simulink model "MARS"  (R2022a)
settings: Solver=VariableStepAuto  StartTime=0.0  StopTime=inf  RelTol=1e-3
model workspace (MAT data in the model file):
  T0 = -23.4
  h_trop = 7
  ingenuityParams.environment.gravity = -3.721
  ingenuityParams.environment.atmDensity = 0.01
  ingenuityParams.mechanical.totalMassExceptBatteries = 1.5
  ingenuityParams.propeller.diameter = 1.2
  ingenuityParams.propeller.inertia = 0.0042
  ingenuityParams.propeller.Jvec = [-0.8 -0.6 -0.4 -0.2 0 0.2 0.4 0.6 0.8 1]
  ingenuityParams.propeller.kTvec = [-0.02 0.02 0.06 0.09 0.12 0.1 0.08 0.05 0 -0.03]
  ingenuityParams.propeller.kPvec = [0.018 0.044 0.055 0.053 0.05 0.051 0.052 0.04 0.015 -0.01]
  ingenuityParams.motordrive.torMax = 0.25
  ingenuityParams.motordrive.powMax = 350
  ingenuityParams.motordrive.Tc = 0.01
  ingenuityParams.motordrive.effRated = 95
  ingenuityParams.motordrive.wRated = 12000
  ingenuityParams.motordrive.torRated = 0.15
  ingenuityParams.motordrive.ironLoss = 1
  ingenuityParams.motordrive.fixedLoss = 0.1
  ingenuityParams.motordrive.supplyRes = 0.07
  ingenuityParams.gearbox.ratio = 5
  ingenuityParams.battery.numSeriesCells = 6
  ingenuityParams.battery.numParallelStrings = 1
  ingenuityParams.battery.numCells = 6
  ingenuityParams.battery.cell.SOCvec = [0 0.01 0.02 0.03 0.04 0.05 0.06 0.07 0.08 0.09 0.1 0.11 0.12 0.13 0.14 0.15 0.16 0.17 0.18 0.19 0.2 0.21 0.22 0.23 0.24 0.25 0.26 0.27 0.28 0.29 0.3 0.31 0.32 0.33 0.34 0.35 0.36 0.37 0.38 0.39 0.4 0.41 0.42 0.43 0.44 0.45 0.46 0.47 0.48 0.49 0.5 0.51 0.52 0.53 0.54 0.55 0.56 0.57 0.58 0.59 0.6 0.61 0.62 0.63 0.64 0.65 0.66 0.67 0.68 0.69 0.7 0.71 0.72 0.73 0.74 0.75 0.76 0.77 0.78 0.79 0.8 0.81 0.82 0.83 0.84 0.85 0.86 0.87 0.88 0.89 0.9 0.91 0.92 0.93 0.94 0.95 0.96 0.97 0.98 0.99 1]
  ingenuityParams.battery.cell.Tvec = [-20 -10 0 20 40]
  ingenuityParams.battery.cell.V0_TLU = [3.43105105188 3.58415322084 3.62260441789 3.64734185538 3.64653306426 3.65558876806 3.66332769116 3.66323970813 3.66627838389 3.66945052656 3.67178851676 3.6762818022 ... (505 elements, 101x5)]
  ingenuityParams.battery.cell.R0_TLU = [0.0677427338002 0.0762862248111 0.0765216743797 0.0757633732548 0.0731538961444 0.0712592375055 0.0700448036528 0.0683159100683 0.0668135859615 0.0653209333694 0.0637678349468 0.0623709173386 ... (505 elements, 101x5)]
  ingenuityParams.battery.cell.AH_TLU = [0.302116721618 0.361031685699 0.377020499472 0.396021549816 0.399328545287]
  ingenuityParams.battery.cell.mass = 0.07
  ingenuityParams.battery.cell.cp = 500
  ingenuityParams.battery.cell.T_init = -16
  ingenuityParams.battery.cell.SOC_init = 0.99
  ingenuityParams.battery.thermal.cell2cellCond.area = 0.0001
  ingenuityParams.battery.thermal.cell2cellCond.thick = 0.01
  ingenuityParams.battery.thermal.cell2cellCond.k = 200
  ingenuityParams.battery.thermal.radToBox.area = 0.00628318530718
  ingenuityParams.battery.thermal.radToBox.radCoeff = 3.969e-08
  ingenuityParams.battery.thermal.insulationLayer.area = 0.24
  ingenuityParams.battery.thermal.insulationLayer.thick = 0.005
  ingenuityParams.battery.thermal.insulationLayer.k = 0.02
  ingenuityParams.battery.thermal.insulantThermalMass.mass = 0.03
  ingenuityParams.battery.thermal.insulantThermalMass.cp = 1200
  ingenuityParams.battery.thermal.radToEnvironment.area = 0.24
  ingenuityParams.battery.thermal.radToEnvironment.radCoeff = 1.701e-08
  ingenuityParams.heater.R = 40
  ingenuityParams.heater.thermalMass = 9
  ingenuityParams.solarcells.Isc = 0.15
  ingenuityParams.solarcells.Voc = 0.85
  ingenuityParams.solarcells.Ir0 = 500
  ingenuityParams.solarcells.qualFactor = 1.5
  ingenuityParams.solarcells.Rs = 0
  ingenuityParams.solarcells.Nseries = 30
  ingenuityParams.solarcells.Nparallel = 1
undefined symbols (not defined in the file): body, collective1, collective2, duration, ingenuity, leg1, leg2, leg3, leg4, link_name, model_name, rotor1, rotor2, solarPanel, world_pose
libraries: fl_lib x35, robotgazebolib x31, nesl_utility x12, ee_lib x11, slpidlib x3, sharedtransform x2, simulink x1, shared6dof x1, aerolibwind2 x1
(part 1 of 3)
settings Model: Creator=aman  LastModifiedBy=aman
settings SolverCC: MaxConsecutiveMinStep=2  ZeroCrossAlgorithm=Adaptive
settings OptimizationCC: DefaultParameterBehavior=Inlined  UseDivisionForNetSlopeComputation=on  GainParamInheritBuiltInType=on  UseFloatMulNetSlope=on  InlineInvariantSignals=on  EfficientFloat2IntCast=on
settings DebuggingCC: IgnoredZcDiagnostic=none
settings HardwareCC: TargetBitPerLong=64  TargetBitPerPointer=64  TargetBitPerSizeT=64  TargetBitPerPtrDiffT=64  TargetLongLongMode=on  TargetIntDivRoundTo=Zero  TargetEndianess=LittleEndian  TargetWordSize=64  TargetHWDeviceType=MATLAB Host  ProdEqTarget=off
settings SFSimCC: MATLABDynamicMemAlloc=off  SimHardwareAcceleration=native  SimTargetLang=C++
settings RTWCC: Description=Rapid Simulation Target  SystemTargetFile=rsim.tlc  TemplateMakefile=rsim_default_tmf  GenerateReport=on  BuildConfiguration=Faster Runs  LaunchReport=on
settings CodeAppCC: ForceParamTrailComments=on
settings RSimTargetCC: TargetLangStandard=C99 (ISO)  OptimizeReductions=off
settings SimscapeCC: SimscapeLogType=all

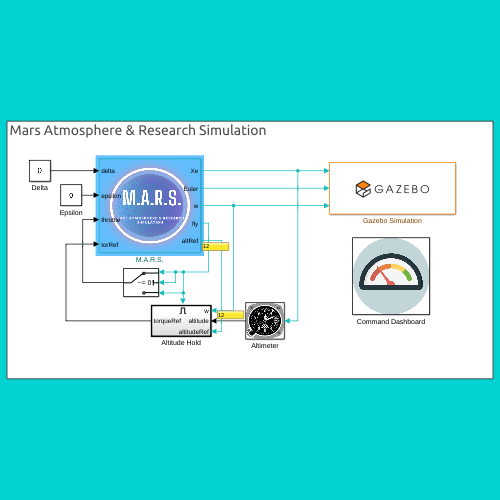
[thumbnail: Simulink's stored preview of the top-level diagram]
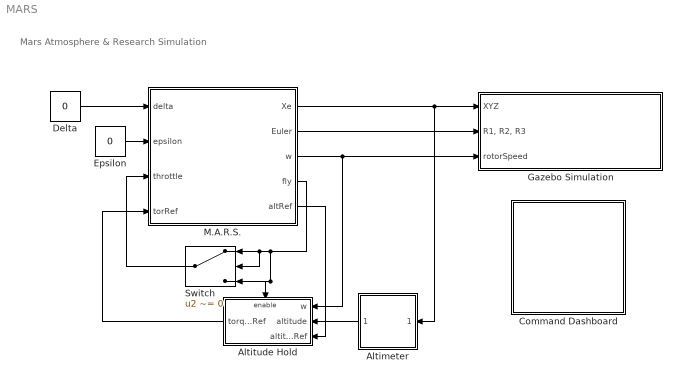
== system MARS ==
  note: Mars Atmosphere & Research Simulation
  Altimeter : Subsystem
      mask Display: image('$imagefile'); % Use "Edit Image" on toolstrip to change.
  Altitude Hold : Subsystem  TreatAsAtomicUnit=on
  Command Dashboard : Subsystem
      mask Display: image('$imagefile'); % Use "Edit Image" on toolstrip to change.
  Delta : Constant  Value=0
  Epsilon : Constant  Value=0
  Gazebo Simulation : Subsystem
      mask Display: image('$imagefile'); % Use "Edit Image" on toolstrip to change.
  M.A.R.S. : Subsystem
      mask Display: image('/home/aman/Desktop/mars.png'); % Use "Edit Image" on toolstrip to change.
  Switch : Switch  Criteria=u2 ~= 0  SaturateOnIntegerOverflow=off  InputSameDT=off
  wires:
  Delta/1 -> M.A.R.S./1(delta)
  Epsilon/1 -> M.A.R.S./2(epsilon)
  M.A.R.S./1(Xe) -> Gazebo Simulation/1(XYZ), Altimeter/1(height)
  Altimeter/1(altitude) -> Altitude Hold/2(altitude)
  M.A.R.S./3(w) -> Gazebo Simulation/3(rotorSpeed), Altitude Hold/1(w)
  Altitude Hold/1(torqueRef) -> M.A.R.S./4(torRef)
  M.A.R.S./5(altRef) -> Altitude Hold/3(altitudeRef)
  M.A.R.S./4(fly) -> Switch/3, Altitude Hold/Enable, Switch/2, Switch/1
  Switch/1 -> M.A.R.S./3(throttle)
  M.A.R.S./2(Euler) -> Gazebo Simulation/2("R1, R2, R3")

== system MARS/Altimeter ==
  height : Inport
  Band-Limited White Noise : simulink/Sources/Band-Limited White Noise  Cov=[0.1]  Ts=0.1  seed=[23341]
  Constant : Constant  Value=0
  Height : MultiPortSwitch  Inputs=1  SaturateOnIntegerOverflow=off  InputSameDT=off
  Index : Constant  Value=3
  Sum : Sum  Inputs=|++
  altitude : Outport
  wires:
  height/1 -> Height/2
  Height/1 -> Sum/2
  Index/1 -> Height/1
  Sum/1 -> altitude/1
  Constant/1 -> Sum/1

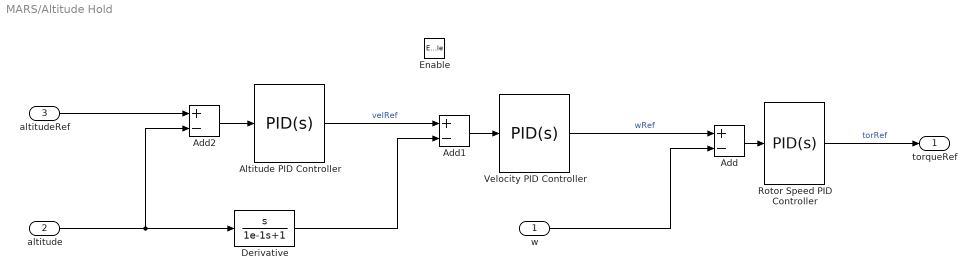
== system MARS/Altitude Hold ==
  w : Inport
  altitude : Inport  Port=2
  altitudeRef : Inport  Port=3
  Enable : EnablePort
  Add : Sum  Inputs=+-
  Add1 : Sum  Inputs=+-
  Add2 : Sum  Inputs=+-
  Altitude PID Controller : slpidlib/PID Controller  Controller=PID  Form=Parallel  TimeDomain=Continuous-time  UseExternalTs=off  SampleTime=-1  IntegratorMethod=Forward Euler  FilterMethod=Forward Euler  ControllerParametersSource=internal  P=2.75291380025279  I=0.654733901603954  UseKiTs=off  D=2.09643844624086  N=374.082600822232  UseFilter=on  TunerSelectOption=Transfer Function Based (PID Tuner App)  ZeroCross=off  InitialConditionSource=internal  InitialConditionForIntegrator=0  InitialConditionForFilter=0  DifferentiatorICPrevScaledInput=0  ExternalReset=none  TrackingMode=off  Kt=1  LimitOutput=on  SatLimitsSource=internal  UpperSaturationLimit=3  LowerSaturationLimit=-3  LinearizeAsGain=off  AntiWindupMode=clamping  Kb=1  POutMin=[]  POutMax=[]  IOutMin=[]  IOutMax=[]  DOutMin=[]  DOutMax=[]  NOutMin=[]  NOutMax=[]  SumOutMin=[]  SumOutMax=[]  SaturationOutMin=[]  SaturationOutMax=[]  PParamMin=[]  PParamMax=[]  IParamMin=[]  IParamMax=[]  DParamMin=[]  DParamMax=[]  NParamMin=[]  NParamMax=[]  KbParamMin=[]  KbParamMax=[]  KtParamMin=[]  KtParamMax=[]  KbOutMin=[]  KbOutMax=[]  KtOutMin=[]  KtOutMax=[]  IntegratorOutMin=[]  IntegratorOutMax=[]  FilterOutMin=[]  FilterOutMax=[]  SumI1OutMin=[]  SumI1OutMax=[]  SumI2OutMin=[]  SumI2OutMax=[]  SumI3OutMin=[]  SumI3OutMax=[]  SumI4OutMin=[]  SumI4OutMax=[]  SumDOutMin=[]  SumDOutMax=[]  DifferentiatorOutMin=[]  DifferentiatorOutMax=[]  FilterDiffOutCoefMin=[]  FilterDiffOutCoefMax=[]  ReciprocalOutMin=[]  ReciprocalOutMax=[]  SumDenOutMin=[]  SumDenOutMax=[]  SumNumOutMin=[]  SumNumOutMax=[]  DivideOutMin=[]  DivideOutMax=[]  UdiffTsProdOutMin=[]  UdiffTsProdOutMax=[]  NTsProdOutMin=[]  NTsProdOutMax=[]  UintegralTsProdOutMin=[]  UintegralTsProdOutMax=[]  UngainTsProdOutMin=[]  UngainTsProdOutMax=[]  IntegratorContinuousStateAttributes=''  IntegratorStateMustResolveToSignalObject=off  IntegratorRTWStateStorageClass=Auto  FilterContinuousStateAttributes=''  FilterStateMustResolveToSignalObject=off  FilterRTWStateStorageClass=Auto  ParallelPVariant=InternalParameters  IdealPVariant=Disabled  IVariant=InternalParameters  DVariant=InternalParameters  IntegratorVariant=Continuous  SatVariant=Enabled  AWVariant=ContClampingParallel  PCopyVariant=Disabled  TRVariant=Disabled  FdbkBlocksVariant=Forward  IdealPFdbkVariant=Disabled  SatFdbkVariant=Disabled  DerivativeFilterVariant=ContFilter  NVariant=InternalParameters  NCopyVariant=Disabled  FilterICVariant=InternalICsFilter  IntegratorICVariant=InternalICs  ExternalResetVariant=Disabled  TRSumVariant=Passthrough  SumFdbkVariant=Disabled  SumVariant=Sum_PID  TsampFilterVariant=InternalTs  TsampNgainVariant=Passthrough  TsampIntegralVariant=Passthrough  ExternalSaturationOutDataTypeStr=Inherit: Same as second input  aMode=0
  Derivative : TransferFcn  Numerator=[1 0]  Denominator=[1e-1 1]
  Rotor Speed PID Controller : slpidlib/PID Controller  Controller=PID  Form=Parallel  TimeDomain=Continuous-time  UseExternalTs=off  SampleTime=-1  IntegratorMethod=Forward Euler  FilterMethod=Forward Euler  ControllerParametersSource=internal  P=0.0108155264440049  I=0.00620055806015913  UseKiTs=off  D=0.000544690366654068  N=7717.3085682068  UseFilter=on  TunerSelectOption=Transfer Function Based (PID Tuner App)  ZeroCross=off  InitialConditionSource=internal  InitialConditionForIntegrator=0  InitialConditionForFilter=0  DifferentiatorICPrevScaledInput=0  ExternalReset=none  TrackingMode=off  Kt=1  LimitOutput=on  SatLimitsSource=internal  UpperSaturationLimit=0.3  LowerSaturationLimit=-0.3  LinearizeAsGain=off  AntiWindupMode=clamping  Kb=1  POutMin=[]  POutMax=[]  IOutMin=[]  IOutMax=[]  DOutMin=[]  DOutMax=[]  NOutMin=[]  NOutMax=[]  SumOutMin=[]  SumOutMax=[]  SaturationOutMin=[]  SaturationOutMax=[]  PParamMin=[]  PParamMax=[]  IParamMin=[]  IParamMax=[]  DParamMin=[]  DParamMax=[]  NParamMin=[]  NParamMax=[]  KbParamMin=[]  KbParamMax=[]  KtParamMin=[]  KtParamMax=[]  KbOutMin=[]  KbOutMax=[]  KtOutMin=[]  KtOutMax=[]  IntegratorOutMin=[]  IntegratorOutMax=[]  FilterOutMin=[]  FilterOutMax=[]  SumI1OutMin=[]  SumI1OutMax=[]  SumI2OutMin=[]  SumI2OutMax=[]  SumI3OutMin=[]  SumI3OutMax=[]  SumI4OutMin=[]  SumI4OutMax=[]  SumDOutMin=[]  SumDOutMax=[]  DifferentiatorOutMin=[]  DifferentiatorOutMax=[]  FilterDiffOutCoefMin=[]  FilterDiffOutCoefMax=[]  ReciprocalOutMin=[]  ReciprocalOutMax=[]  SumDenOutMin=[]  SumDenOutMax=[]  SumNumOutMin=[]  SumNumOutMax=[]  DivideOutMin=[]  DivideOutMax=[]  UdiffTsProdOutMin=[]  UdiffTsProdOutMax=[]  NTsProdOutMin=[]  NTsProdOutMax=[]  UintegralTsProdOutMin=[]  UintegralTsProdOutMax=[]  UngainTsProdOutMin=[]  UngainTsProdOutMax=[]  IntegratorContinuousStateAttributes=''  IntegratorStateMustResolveToSignalObject=off  IntegratorRTWStateStorageClass=Auto  FilterContinuousStateAttributes=''  FilterStateMustResolveToSignalObject=off  FilterRTWStateStorageClass=Auto  ParallelPVariant=InternalParameters  IdealPVariant=Disabled  IVariant=InternalParameters  DVariant=InternalParameters  IntegratorVariant=Continuous  SatVariant=Enabled  AWVariant=ContClampingParallel  PCopyVariant=Disabled  TRVariant=Disabled  FdbkBlocksVariant=Forward  IdealPFdbkVariant=Disabled  SatFdbkVariant=Disabled  DerivativeFilterVariant=ContFilter  NVariant=InternalParameters  NCopyVariant=Disabled  FilterICVariant=InternalICsFilter  IntegratorICVariant=InternalICs  ExternalResetVariant=Disabled  TRSumVariant=Passthrough  SumFdbkVariant=Disabled  SumVariant=Sum_PID  TsampFilterVariant=InternalTs  TsampNgainVariant=Passthrough  TsampIntegralVariant=Passthrough  ExternalSaturationOutDataTypeStr=Inherit: Same as second input  aMode=0
  Velocity PID Controller : slpidlib/PID Controller  Controller=PID  Form=Parallel  TimeDomain=Continuous-time  UseExternalTs=off  SampleTime=-1  IntegratorMethod=Forward Euler  FilterMethod=Forward Euler  ControllerParametersSource=internal  P=155.19306060889  I=41.1553609138668  UseKiTs=off  D=46.7041807942439  N=1.30346385486406  UseFilter=on  TunerSelectOption=Transfer Function Based (PID Tuner App)  ZeroCross=off  InitialConditionSource=internal  InitialConditionForIntegrator=0  InitialConditionForFilter=0  DifferentiatorICPrevScaledInput=0  ExternalReset=none  TrackingMode=off  Kt=1  LimitOutput=on  SatLimitsSource=internal  UpperSaturationLimit=1600  LowerSaturationLimit=0  LinearizeAsGain=off  AntiWindupMode=clamping  Kb=1  POutMin=[]  POutMax=[]  IOutMin=[]  IOutMax=[]  DOutMin=[]  DOutMax=[]  NOutMin=[]  NOutMax=[]  SumOutMin=[]  SumOutMax=[]  SaturationOutMin=[]  SaturationOutMax=[]  PParamMin=[]  PParamMax=[]  IParamMin=[]  IParamMax=[]  DParamMin=[]  DParamMax=[]  NParamMin=[]  NParamMax=[]  KbParamMin=[]  KbParamMax=[]  KtParamMin=[]  KtParamMax=[]  KbOutMin=[]  KbOutMax=[]  KtOutMin=[]  KtOutMax=[]  IntegratorOutMin=[]  IntegratorOutMax=[]  FilterOutMin=[]  FilterOutMax=[]  SumI1OutMin=[]  SumI1OutMax=[]  SumI2OutMin=[]  SumI2OutMax=[]  SumI3OutMin=[]  SumI3OutMax=[]  SumI4OutMin=[]  SumI4OutMax=[]  SumDOutMin=[]  SumDOutMax=[]  DifferentiatorOutMin=[]  DifferentiatorOutMax=[]  FilterDiffOutCoefMin=[]  FilterDiffOutCoefMax=[]  ReciprocalOutMin=[]  ReciprocalOutMax=[]  SumDenOutMin=[]  SumDenOutMax=[]  SumNumOutMin=[]  SumNumOutMax=[]  DivideOutMin=[]  DivideOutMax=[]  UdiffTsProdOutMin=[]  UdiffTsProdOutMax=[]  NTsProdOutMin=[]  NTsProdOutMax=[]  UintegralTsProdOutMin=[]  UintegralTsProdOutMax=[]  UngainTsProdOutMin=[]  UngainTsProdOutMax=[]  IntegratorContinuousStateAttributes=''  IntegratorStateMustResolveToSignalObject=off  IntegratorRTWStateStorageClass=Auto  FilterContinuousStateAttributes=''  FilterStateMustResolveToSignalObject=off  FilterRTWStateStorageClass=Auto  ParallelPVariant=InternalParameters  IdealPVariant=Disabled  IVariant=InternalParameters  DVariant=InternalParameters  IntegratorVariant=Continuous  SatVariant=Enabled  AWVariant=ContClampingParallel  PCopyVariant=Disabled  TRVariant=Disabled  FdbkBlocksVariant=Forward  IdealPFdbkVariant=Disabled  SatFdbkVariant=Disabled  DerivativeFilterVariant=ContFilter  NVariant=InternalParameters  NCopyVariant=Disabled  FilterICVariant=InternalICsFilter  IntegratorICVariant=InternalICs  ExternalResetVariant=Disabled  TRSumVariant=Passthrough  SumFdbkVariant=Disabled  SumVariant=Sum_PID  TsampFilterVariant=InternalTs  TsampNgainVariant=Passthrough  TsampIntegralVariant=Passthrough  ExternalSaturationOutDataTypeStr=Inherit: Same as second input  aMode=0
  torqueRef : Outport  OutputWhenDisabled=reset  InitialOutput=0
  wires:
  Add2/1 -> Altitude PID Controller/1
  Rotor Speed PID Controller/1 -> torqueRef/1  "torRef"
  Add/1 -> Rotor Speed PID Controller/1
  Add1/1 -> Velocity PID Controller/1
  w/1 -> Add/2
  Velocity PID Controller/1 -> Add/1  "wRef"
  altitude/1 -> Add2/2, Derivative/1
  Derivative/1 -> Add1/2
  Altitude PID Controller/1 -> Add1/1  "velRef"
  altitudeRef/1 -> Add2/1

== system MARS/Command Dashboard ==
  note: Measurements and Controller State
  note: Martian Environment Variables & Controls
  Altimeter : AltimeterBlock
  Altitude [m] : LinearGaugeBlock  LabelPosition=Hide  ScaleMax=50  TickInterval=2
  Artificial Horizon : ArtificialHorizonBlock
  Battery SOC : CircularGaugeBlock  LabelPosition=Hide  ScaleMax=1  TickInterval=0.2
  "Battery Temperature [degC] " : SemiCircularGaugeBlock  LabelPosition=Hide  ScaleMin=-60  ScaleMax=40  TickInterval=20
  Flying : LampBlock  LabelPosition=Hide
  Heater On : LampBlock  LabelPosition=Hide
  Prepare Flight : ToggleSwitchBlock  LabelPosition=Hide
      settings: Values={{'Off', 'On'}, [0 1]}
  Solar Irradiation [W/m^2] : SliderBlock  LabelPosition=Hide  ScaleMax=500
  Surface Temperature [degC] : SliderBlock  LabelPosition=Hide  ScaleMin=-125  ScaleMax=50
  delta : CustomTuningWebBlock  LabelPosition=Hide  ShowInitialText=on  Configuration="{\"type\":\"LinearGauge\",\"settings\":{\"BindingType\":\"param\",\"aspectRatio\":3.7777777777777777,\"backgroundColor\":[0,0,0,\"1\"],\"backgroundOffset\":0,\"backgroundOpacity\":1,\"fixedAspectRatio\":\"on\",\"foregroundColor\":[252,252,196],\"orientation\":\"horizontal\",\"showBackgroundColor\":false,\"value\":0},\"components\":[{\"name\":\"LinearScaleComponent\",\"settings\":{\"bounds\":{\"max\":0.1,\"min\":-0.1,\"tickInterval\":\"auto\"},\"internalTickHeightScaleFactor\":0.5,\"labelColor\":[255,255,200],\"labelFont\":{\"font\":\"Arial\",\"fontSize\":12},\"labelTransparency\":1,\"needleImage\":{\"size\":[596,842],\"src\":\"data:image/svg+xml;base64,PD94bWwgdmVyc2lvbj0iMS4wIiBlbmNvZGluZz0idXRmLTgiPz4NCjwhLS0gR2VuZXJhdG9yOiBBZG9iZSBJbGx1c3RyYXRvciAyNS4wLjAsIFNWRyBFeHBvcnQgUGx1Zy1JbiAuIFNWRyBWZXJzaW9uOiA2LjAwIEJ1aWxkIDApICAtLT4NCjxzdmcgdmVyc2lvbj0iMS4xIg0KCSBpZD0ic3ZnOCIgeG1sbnM6Y2M9Imh0dHA6Ly9jcmVhdGl2ZWNvbW1vbnMub3JnL25zIyIgeG1sbnM6ZGM9Imh0dHA6Ly9wdXJsLm9yZy9kYy9lbGVtZW50cy8xLjEvIiB4bWxuczppbmtzY2FwZT0iaHR0cDovL3d3dy5pbmtzY2FwZS5vcmcvbmFtZXNw ...(+2420 chars)\",\"srcOrientation\":\"horizontal\"},\"needleOffset\":[-0.8044596912521441,-0.0642123287671233],\"needleSize\":{\"height\":0.4337797619047619,\"width\":0.07668067226890757},\"position\":[0.2829861111111111,0.04398634453781513,0.9196428571428571,0.6088789682539683],\"referencePoint\":\"auto\",\"scaleColors\":[],\"scaleColorsSize\":0.2,\"scaleDirection\":\"LR\",\"showLabels\":1,\"showMinorTicks\":0,\"showSpanLine\":1,\"showTicks\":1,\"tickColor\":[252,252,197],\"tickTransparency\":1,\"valueBarColor\":[0,114,189],\"valueBarOffset\":-0.27,\"valueBarSize\":0.1,\"valueBarTransparency\":1}},{\"name\":\"BackgroundImageComponent\",\"settings\":{\"image\":{\"size\":[380,101],\"src\":\"data:image/svg+xml;base64,PHN2ZyB4bWxucz0iaHR0cDovL3d3dy53My5vcmcvMjAwMC9zdmciIHhtbG5zOnhsaW5rPSJodHRwOi8vd3d3LnczLm9yZy8xOTk5L3hsaW5rIiB2aWV3Qm94PSIwIDAgMzgwIDEwMSI+PGRlZnM+PHN0eWxlPi5jbHMtMXtmaWxsOiMwMDJiNDI7fS5jbHMtMntmaWxsOiM0MjcwODI7fS5jbHMtM3tmaWxsOnVybCgjcmFkaWFsLWdyYWRpZW50KTt9LmNscy00e2ZpbGw6I2M4YzhjODtzdHJva2U6IzAwMDt9PC9zdHlsZT48cmFkaWFsR3JhZGllbnQgaWQ9InJhZGlhbC1ncmFkaWVudCIgY3g9IjE5MCIgY3k9IjUwLjUiIHI9IjI2OS4yMSIgZ3JhZGllbnRVbml0cz0idXNlclNwYWNlT25Vc2UiPjxzdG9wIG9mZnNldD0iMC4wMSIgc3RvcC1jb2xvcj0iIzNlNGY1OCIvPjxzdG9wIG9mZnNldD0iMC4wNiIgc3RvcC1jb2xvcj0iIzQ0NTc2MSIvPjxzdG9wIG9mZnNldD0iMC4xNSIgc3RvcC1jb2xvcj0iIzU1NmE3NiIvPjxzdG9wIG9mZnNldD0iMC4yNSIgc3RvcC1jb2xvcj0iIzZkODg5NSIvPjxzdG9wIG9mZnNldD0iMC4zOCIgc3RvcC1jb2xvcj0iIzhmYjJjMyIvPjxzdG9wIG9mZnNldD0iMC41MiIgc3RvcC1jb2xvcj0iI2I2ZTRmYSIvPjxzdG9wIG9mZnNldD0iMSIgc3RvcC1jb2xvcj0iIzE1NDY1NyIvPjwvcmFkaWFsR3JhZGllbnQ+PC9kZWZzPjxnIGlkPSJmcmFtZSI+PGcgaWQ9IkxheWVyXzIiIGRhdGEtbmFtZT0iTGF5ZXIgMiI+PGcgaWQ9IkxheWVyXzEtMiIgZGF0YS1uYW1lPSJMYXllciAxLTIiPjxyZWN0IGlkPSJyZWN0MTAzNiIgY2xhc3M9ImNscy0xIiB4PSIxMSIgeT0iMTEiIHdpZHRoPSIzNTgiIGhlaWdodD0iNzkiLz48cGF0aCBpZD0icGF0aDEwMzgiIGNsYXNzPSJjbHMtMiIgZD0iTTgsOFY5M0gzNzJWOFpNMzY5LDkwSDExVjExSDM2OVoiLz48cGF0aCBpZD0icGF0aDEwNDAiIGNsYXNzPSJjbHMtMyIgZD0iTTAsMFYxMDFIMzgwVjBaTTM3Miw5M0g4VjhIMzcyWiIvPjwvZz48L2c+PC9nPjxnIGlkPSJ0cmFjayI+PHBhdGggaWQ9InJlY3QxNjExIiBjbGFzcz0iY2xzLTQiIGQ9Ik0zMy4zNywyNi41OUgzNDYuNjNjNCwwLDcuMjUsMi42LDcuMjUsNS44MWgwYzAsMy4yMS0zLjI1LDUuODItNy4yNSw1LjgySDMzLjM3Yy00LDAtNy4yNS0yLjYxLTcuMjUtNS44MmgwQzI2LjEyLDI5LjE5LDI5LjM3LDI2LjU5LDMzLjM3LDI2LjU5WiIvPjwvZz48L3N2Zz4=\",\"srcOrientation\":\"horizontal\"},\"position\":[0,0,1,1],\"scaleMode\":\"0\"}},{\"name\":\"ForegroundImageComponent\",\"settings\":{\"image\":{\"size\":[0,0],\"src\":\"default\",\"srcOrientation\":[]},\"isForeground\":1,\"position\":[0,0,1,1],\"scaleMode\":\"0\"}}]}"
  epsilon : CustomTuningWebBlock  LabelPosition=Hide  ShowInitialText=on  Configuration="{\"type\":\"LinearGauge\",\"settings\":{\"BindingType\":\"param\",\"aspectRatio\":3.7777777777777777,\"backgroundColor\":[0,0,0,\"1\"],\"backgroundOffset\":0,\"backgroundOpacity\":1,\"fixedAspectRatio\":\"on\",\"foregroundColor\":[252,252,196],\"orientation\":\"horizontal\",\"showBackgroundColor\":false,\"value\":0},\"components\":[{\"name\":\"LinearScaleComponent\",\"settings\":{\"bounds\":{\"max\":6.28,\"min\":0,\"tickInterval\":\"auto\"},\"internalTickHeightScaleFactor\":0.5,\"labelColor\":[255,255,200],\"labelFont\":{\"font\":\"Arial\",\"fontSize\":12},\"labelTransparency\":1,\"needleImage\":{\"size\":[596,842],\"src\":\"data:image/svg+xml;base64,PD94bWwgdmVyc2lvbj0iMS4wIiBlbmNvZGluZz0idXRmLTgiPz4NCjwhLS0gR2VuZXJhdG9yOiBBZG9iZSBJbGx1c3RyYXRvciAyNS4wLjAsIFNWRyBFeHBvcnQgUGx1Zy1JbiAuIFNWRyBWZXJzaW9uOiA2LjAwIEJ1aWxkIDApICAtLT4NCjxzdmcgdmVyc2lvbj0iMS4xIg0KCSBpZD0ic3ZnOCIgeG1sbnM6Y2M9Imh0dHA6Ly9jcmVhdGl2ZWNvbW1vbnMub3JnL25zIyIgeG1sbnM6ZGM9Imh0dHA6Ly9wdXJsLm9yZy9kYy9lbGVtZW50cy8xLjEvIiB4bWxuczppbmtzY2FwZT0iaHR0cDovL3d3dy5pbmtzY2FwZS5vcmcvbmFtZXNw ...(+2420 chars)\",\"srcOrientation\":\"horizontal\"},\"needleOffset\":[-0.8044596912521441,-0.0642123287671233],\"needleSize\":{\"height\":0.4337797619047619,\"width\":0.07668067226890757},\"position\":[0.2829861111111111,0.04398634453781513,0.9196428571428571,0.6088789682539683],\"referencePoint\":\"auto\",\"scaleColors\":[],\"scaleColorsSize\":0.2,\"scaleDirection\":\"LR\",\"showLabels\":1,\"showMinorTicks\":0,\"showSpanLine\":1,\"showTicks\":1,\"tickColor\":[252,252,197],\"tickTransparency\":1,\"valueBarColor\":[0,114,189],\"valueBarOffset\":-0.27,\"valueBarSize\":0.1,\"valueBarTransparency\":1}},{\"name\":\"BackgroundImageComponent\",\"settings\":{\"image\":{\"size\":[380,101],\"src\":\"data:image/svg+xml;base64,PHN2ZyB4bWxucz0iaHR0cDovL3d3dy53My5vcmcvMjAwMC9zdmciIHhtbG5zOnhsaW5rPSJodHRwOi8vd3d3LnczLm9yZy8xOTk5L3hsaW5rIiB2aWV3Qm94PSIwIDAgMzgwIDEwMSI+PGRlZnM+PHN0eWxlPi5jbHMtMXtmaWxsOiMwMDJiNDI7fS5jbHMtMntmaWxsOiM0MjcwODI7fS5jbHMtM3tmaWxsOnVybCgjcmFkaWFsLWdyYWRpZW50KTt9LmNscy00e2ZpbGw6I2M4YzhjODtzdHJva2U6IzAwMDt9PC9zdHlsZT48cmFkaWFsR3JhZGllbnQgaWQ9InJhZGlhbC1ncmFkaWVudCIgY3g9IjE5MCIgY3k9IjUwLjUiIHI9IjI2OS4yMSIgZ3JhZGllbnRVbml0cz0idXNlclNwYWNlT25Vc2UiPjxzdG9wIG9mZnNldD0iMC4wMSIgc3RvcC1jb2xvcj0iIzNlNGY1OCIvPjxzdG9wIG9mZnNldD0iMC4wNiIgc3RvcC1jb2xvcj0iIzQ0NTc2MSIvPjxzdG9wIG9mZnNldD0iMC4xNSIgc3RvcC1jb2xvcj0iIzU1NmE3NiIvPjxzdG9wIG9mZnNldD0iMC4yNSIgc3RvcC1jb2xvcj0iIzZkODg5NSIvPjxzdG9wIG9mZnNldD0iMC4zOCIgc3RvcC1jb2xvcj0iIzhmYjJjMyIvPjxzdG9wIG9mZnNldD0iMC41MiIgc3RvcC1jb2xvcj0iI2I2ZTRmYSIvPjxzdG9wIG9mZnNldD0iMSIgc3RvcC1jb2xvcj0iIzE1NDY1NyIvPjwvcmFkaWFsR3JhZGllbnQ+PC9kZWZzPjxnIGlkPSJmcmFtZSI+PGcgaWQ9IkxheWVyXzIiIGRhdGEtbmFtZT0iTGF5ZXIgMiI+PGcgaWQ9IkxheWVyXzEtMiIgZGF0YS1uYW1lPSJMYXllciAxLTIiPjxyZWN0IGlkPSJyZWN0MTAzNiIgY2xhc3M9ImNscy0xIiB4PSIxMSIgeT0iMTEiIHdpZHRoPSIzNTgiIGhlaWdodD0iNzkiLz48cGF0aCBpZD0icGF0aDEwMzgiIGNsYXNzPSJjbHMtMiIgZD0iTTgsOFY5M0gzNzJWOFpNMzY5LDkwSDExVjExSDM2OVoiLz48cGF0aCBpZD0icGF0aDEwNDAiIGNsYXNzPSJjbHMtMyIgZD0iTTAsMFYxMDFIMzgwVjBaTTM3Miw5M0g4VjhIMzcyWiIvPjwvZz48L2c+PC9nPjxnIGlkPSJ0cmFjayI+PHBhdGggaWQ9InJlY3QxNjExIiBjbGFzcz0iY2xzLTQiIGQ9Ik0zMy4zNywyNi41OUgzNDYuNjNjNCwwLDcuMjUsMi42LDcuMjUsNS44MWgwYzAsMy4yMS0zLjI1LDUuODItNy4yNSw1LjgySDMzLjM3Yy00LDAtNy4yNS0yLjYxLTcuMjUtNS44MmgwQzI2LjEyLDI5LjE5LDI5LjM3LDI2LjU5LDMzLjM3LDI2LjU5WiIvPjwvZz48L3N2Zz4=\",\"srcOrientation\":\"horizontal\"},\"position\":[0,0,1,1],\"scaleMode\":\"0\"}},{\"name\":\"ForegroundImageComponent\",\"settings\":{\"image\":{\"size\":[0,0],\"src\":\"default\",\"srcOrientation\":[]},\"isForeground\":1,\"position\":[0,0,1,1],\"scaleMode\":\"0\"}}]}"

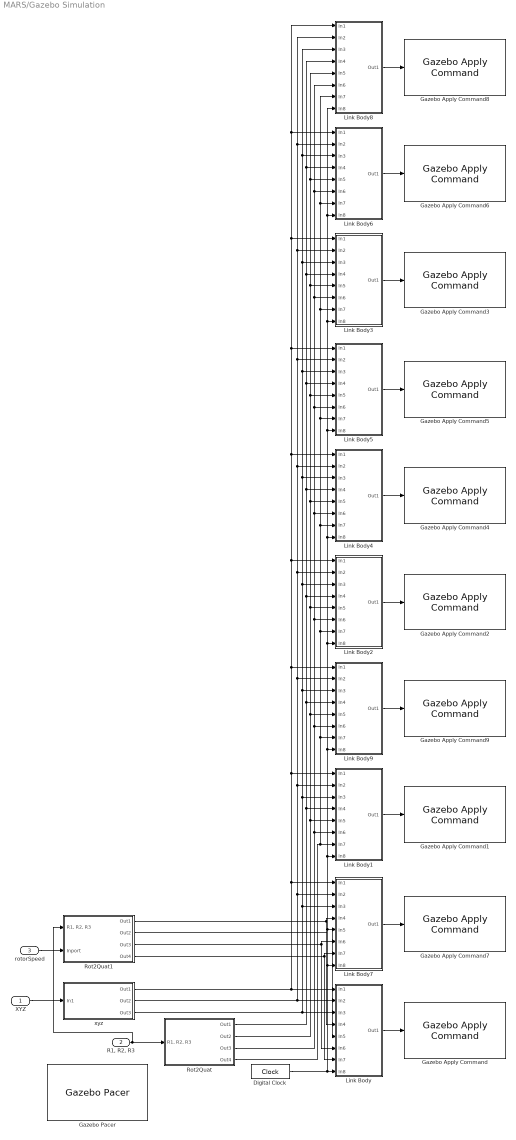
== system MARS/Gazebo Simulation ==
  XYZ : Inport
  "R1, R2, R3" : Inport  Port=2
  rotorSpeed : Inport  Port=3
  Digital Clock : DigitalClock  SampleTime=0.01
  Gazebo Apply Command{,1..9} (10 alike) : robotgazebolib/Gazebo Apply Command  cmdType=SetLinkWorldPose  sampleTime=0.01
      settings: SourceProductBaseCode=RO
  Gazebo Pacer : robotgazebolib/Gazebo Pacer  ResetBehavior=Reset Gazebo simulation time and scene  SampleTime=0.01
      settings: SourceProductBaseCode=RO
  Link Body : Subsystem
  Link Body1 : Subsystem
  Link Body2 : Subsystem
  Link Body3 : Subsystem
  Link Body4 : Subsystem
  Link Body5 : Subsystem
  Link Body6 : Subsystem
  Link Body7 : Subsystem
  Link Body8 : Subsystem
  Link Body9 : Subsystem
  Rot2Quat : Subsystem
  Rot2Quat1 : Subsystem
  xyz : Subsystem
  wires:
  XYZ/1 -> xyz/1(In1)
  xyz/2(Out2) -> Link Body/2(In2), Link Body7/2(In2), Link Body1/2(In2), Link Body9/2(In2), Link Body8/2(In2), Link Body6/2(In2), Link Body3/2(In2), Link Body5/2(In2), Link Body4/2(In2), Link Body2/2(In2)
  "R1, R2, R3"/1 -> Rot2Quat1/1("R1, R2, R3"), Rot2Quat/1("R1, R2, R3")
  Rot2Quat/3(Out3) -> Link Body1/6(In6), Link Body9/6(In6), Link Body2/6(In6), Link Body8/6(In6), Link Body6/6(In6), Link Body3/6(In6), Link Body5/6(In6), Link Body4/6(In6)
  Link Body8/1(Out1) -> Gazebo Apply Command8/1
  Link Body4/1(Out1) -> Gazebo Apply Command4/1
  Link Body2/1(Out1) -> Gazebo Apply Command2/1
  Link Body6/1(Out1) -> Gazebo Apply Command6/1
  Link Body5/1(Out1) -> Gazebo Apply Command5/1
  Link Body3/1(Out1) -> Gazebo Apply Command3/1
  Digital Clock/1 -> Link Body8/8(In8), Link Body6/8(In8), Link Body3/8(In8), Link Body5/8(In8), Link Body4/8(In8), Link Body2/8(In8), Link Body9/8(In8), Link Body1/8(In8), Link Body7/8(In8), Link Body/8(In8)
  Link Body7/1(Out1) -> Gazebo Apply Command7/1
  Link Body1/1(Out1) -> Gazebo Apply Command1/1
  xyz/1(Out1) -> Link Body9/1(In1), Link Body2/1(In1), Link Body4/1(In1), Link Body5/1(In1), Link Body3/1(In1), Link Body6/1(In1), Link Body8/1(In1), Link Body1/1(In1), Link Body7/1(In1), Link Body/1(In1)
  xyz/3(Out3) -> Link Body/3(In3), Link Body7/3(In3), Link Body1/3(In3), Link Body9/3(In3), Link Body8/3(In3), Link Body6/3(In3), Link Body3/3(In3), Link Body5/3(In3), Link Body4/3(In3), Link Body2/3(In3)
  Link Body/1(Out1) -> Gazebo Apply Command/1
  Rot2Quat/2(Out2) -> Link Body1/5(In5), Link Body9/5(In5), Link Body2/5(In5), Link Body6/5(In5), Link Body8/5(In5), Link Body3/5(In5), Link Body5/5(In5), Link Body4/5(In5)
  Link Body9/1(Out1) -> Gazebo Apply Command9/1
  Rot2Quat/4(Out4) -> Link Body1/7(In7), Link Body9/7(In7), Link Body2/7(In7), Link Body3/7(In7), Link Body8/7(In7), Link Body6/7(In7), Link Body5/7(In7), Link Body4/7(In7)
  Rot2Quat/1(Out1) -> Link Body1/4(In4), Link Body9/4(In4), Link Body8/4(In4), Link Body6/4(In4), Link Body3/4(In4), Link Body5/4(In4), Link Body4/4(In4), Link Body2/4(In4)
  Rot2Quat1/1(Out1) -> Link Body7/4(In4), Link Body/4(In4)
  Rot2Quat1/2(Out2) -> Link Body/5(In5), Link Body7/5(In5)
  Rot2Quat1/3(Out3) -> Link Body7/6(In6), Link Body/6(In6)
  Rot2Quat1/4(Out4) -> Link Body7/7(In7), Link Body/7(In7)
  rotorSpeed/1 -> Rot2Quat1/2(Inport)

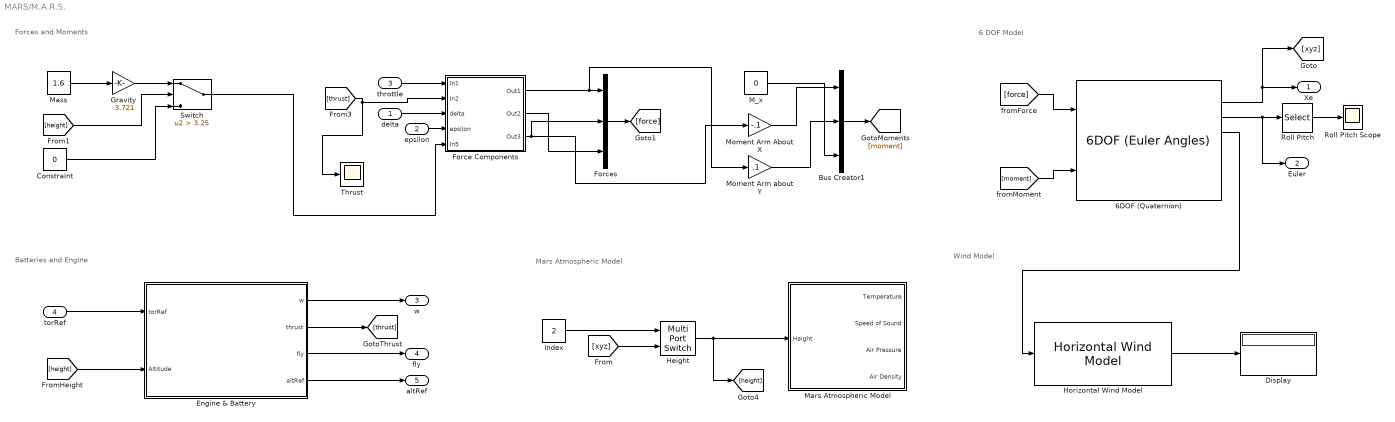
== system MARS/M.A.R.S. ==
  note: Wind Model
  note: Batteries and Engine
  note: Forces and Moments
  note: 6 DOF Model
  note: Mars Atmospheric Model
  delta : Inport
  epsilon : Inport  Port=2
  throttle : Inport  Port=3
  torRef : Inport  Port=4
  6DOF (Quaternion) : shared6dof/6DOF (Euler Angles)  units=Metric (MKS)  mtype=Fixed  rep=Quaternion  xme_0=[0 0 3.2]  Vm_0=[0 0 0]  eul_0=[0 0 0]  pm_0=[0 0 0]  mass_0=1.0  mass_e=0.5  mass_f=2.0  inertia=eye(3)  inertia_e=eye(3)  inertia_f=2*eye(3)  k_quat=1.0  vre_flag=on  abi_flag=off  aMode=0  xme_statename=''  Vm_statename=''  eul_statename=''  quat_statename=''  pm_statename=''  mass_statename=''
      settings: SourceProductBaseCode=AE,PW,DR,MT,VE
  Bus Creator1 : BusCreator  Inputs=3
  Constraint : Constant  Value=0
  Display : Display
  Engine & Battery : Subsystem
      mask Display: image('$imagefile'); % Use "Edit Image" on toolstrip to change.
  Force Components : Subsystem
  Forces : BusCreator  Inputs=3
  Gravity : Gain  Gain=-3.721
  Height : MultiPortSwitch  DataPortOrder=Zero-based contiguous  Inputs=1  zeroidx=on  SaturateOnIntegerOverflow=off  InputSameDT=off
  Horizontal Wind Model : aerolibwind2/Horizontal Wind Model  units=Metric (MKS)  Vw_source=Internal  Vwind=15  W_source=Internal  Wdeg=0
      settings: SourceProductBaseCode=AE
  Index : Constant  Value=2
  M_x : Constant  Value=0
  Mars Atmospheric Model : Subsystem  mask{height_lim=7000, T0=-23.4+273.1, P0=699, TempLapse=-0.000998, PresLapse=-0.00009, Gamma=1.2, R=192.1}
      mask prompts: height_lim "Max Height"; T0 "Temperature At Surface"; P0 "Pressure At Surface"; TempLapse "Temperature Lapse"; PresLapse "Pressure Lapse"; R "Gas Constant"
      mask Display: image('$imagefile'); % Use "Edit Image" on toolstrip to change.
  Mass : Constant  Value=1.6
  Moment Arm About X : Gain  Gain=-.1
  Moment Arm about Y : Gain  Gain=.1
  Roll Pitch : Selector  InputPortWidth=3  IndexOptions=Index vector (dialog)  Indices=[1 2]  OutputSizes=1
  Roll Pitch Scope : Scope
  Switch : Switch  Criteria=u2 > Threshold  Threshold=3.25  SaturateOnIntegerOverflow=off  InputSameDT=off
  Thrust : Scope
  Xe : Outport
  Euler : Outport  Port=2
  w : Outport  Port=3
  fly : Outport  Port=4
  altRef : Outport  Port=5
  wires:
  6DOF (Quaternion)/2 -> [xyz], Xe/1
  Index/1 -> Height/1
  Mass/1 -> Gravity/1
  Height/1 -> Mars Atmospheric Model/1(Height), [height]
  [xyz] -> Height/2
  Forces/1 -> [force]
  [force] -> 6DOF (Quaternion)/1
  Bus Creator1/1 -> [moment]
  [moment] -> 6DOF (Quaternion)/2
  Engine & Battery/1(w) -> w/1
  torRef/1 -> Engine & Battery/1(torRef)
  [height] -> Engine & Battery/2(Altitude)
  Engine & Battery/3(fly) -> fly/1
  Engine & Battery/4(altRef) -> altRef/1
  Constraint/1 -> Switch/3
  Gravity/1 -> Switch/1
  [height] -> Switch/2
  Engine & Battery/2(thrust) -> [thrust]
  Force Components/3(Out3) -> Forces/2, Moment Arm About X/1
  Force Components/1(Out1) -> Moment Arm about Y/1, Forces/1
  throttle/1 -> Force Components/1(In1)
  delta/1 -> Force Components/3(delta)
  epsilon/1 -> Force Components/4(epsilon)
  Switch/1 -> Force Components/5(In5)
  [thrust] -> Force Components/2(In2), Thrust/1
  6DOF (Quaternion)/3 -> Roll Pitch/1, Euler/1
  Roll Pitch/1 -> Roll Pitch Scope/1
  Horizontal Wind Model/1 -> Display/1
  6DOF (Quaternion)/4 -> Horizontal Wind Model/1
  Moment Arm About X/1 -> Bus Creator1/1
  Moment Arm about Y/1 -> Bus Creator1/2
  M_x/1 -> Bus Creator1/3
  Force Components/2(Out2) -> Forces/3

== system MARS/Gazebo Simulation/Link Body ==
  In1 : Inport
  In2 : Inport  Port=2
  In3 : Inport  Port=3
  In4 : Inport  Port=4
  In5 : Inport  Port=5
  In6 : Inport  Port=6
  In7 : Inport  Port=7
  In8 : Inport  Port=8
  Bus Assignment : BusAssignment  AssignedSignals=model_name,link_name,world_pose.position.x,world_pose.position.y,world_pose.position.z,world_pose.orientation.w,world_pose.orientation.x,world_pose.orientation.y,world_pose.orientation.z,duration.seconds
  Gazebo Blank Message : robotgazebolib/Gazebo Blank Message  msgType=SetLinkWorldPose  sampleTime=0.01  busName='Gazebo_SL_Bus_gazebo_msgs_SetLinkWorldPose'
      settings: SourceProductBaseCode=RO
  Gazebo Select Entity : robotgazebolib/Gazebo Select Entity  modelElemName=ingenuity/rotor2  outputArraySize=128  OutputLabel=Link  SelectType=Link
      settings: SourceProductBaseCode=RO
  Out1 : Outport
  wires:
  In6/1 -> Bus Assignment/9
  In4/1 -> Bus Assignment/7
  In3/1 -> Bus Assignment/6
  In7/1 -> Bus Assignment/10
  In2/1 -> Bus Assignment/5
  Bus Assignment/1 -> Out1/1
  Gazebo Select Entity/2 -> Bus Assignment/3
  In5/1 -> Bus Assignment/8
  Gazebo Blank Message/1 -> Bus Assignment/1
  In8/1 -> Bus Assignment/11
  In1/1 -> Bus Assignment/4
  Gazebo Select Entity/1 -> Bus Assignment/2

== system MARS/Gazebo Simulation/Link Body1 ==
  In1 : Inport
  In2 : Inport  Port=2
  In3 : Inport  Port=3
  In4 : Inport  Port=4
  In5 : Inport  Port=5
  In6 : Inport  Port=6
  In7 : Inport  Port=7
  In8 : Inport  Port=8
  Bus Assignment : BusAssignment  AssignedSignals=model_name,link_name,world_pose.position.x,world_pose.position.y,world_pose.position.z,world_pose.orientation.w,world_pose.orientation.x,world_pose.orientation.y,world_pose.orientation.z,duration.seconds
  Gazebo Blank Message : robotgazebolib/Gazebo Blank Message  msgType=SetLinkWorldPose  sampleTime=0.01  busName='Gazebo_SL_Bus_gazebo_msgs_SetLinkWorldPose'
      settings: SourceProductBaseCode=RO
  Gazebo Select Entity : robotgazebolib/Gazebo Select Entity  modelElemName=ingenuity/solarPanel  outputArraySize=128  OutputLabel=Link  SelectType=Link
      settings: SourceProductBaseCode=RO
  Out1 : Outport
  wires:
  Gazebo Select Entity/1 -> Bus Assignment/2
  In1/1 -> Bus Assignment/4
  In8/1 -> Bus Assignment/11
  Gazebo Blank Message/1 -> Bus Assignment/1
  In5/1 -> Bus Assignment/8
  Gazebo Select Entity/2 -> Bus Assignment/3
  Bus Assignment/1 -> Out1/1
  In2/1 -> Bus Assignment/5
  In7/1 -> Bus Assignment/10
  In3/1 -> Bus Assignment/6
  In4/1 -> Bus Assignment/7
  In6/1 -> Bus Assignment/9

== system MARS/Gazebo Simulation/Link Body2 ==
  In1 : Inport
  In2 : Inport  Port=2
  In3 : Inport  Port=3
  In4 : Inport  Port=4
  In5 : Inport  Port=5
  In6 : Inport  Port=6
  In7 : Inport  Port=7
  In8 : Inport  Port=8
  Bus Assignment : BusAssignment  AssignedSignals=model_name,link_name,world_pose.position.x,world_pose.position.y,world_pose.position.z,world_pose.orientation.w,world_pose.orientation.x,world_pose.orientation.y,world_pose.orientation.z,duration.seconds
  Gazebo Blank Message : robotgazebolib/Gazebo Blank Message  msgType=SetLinkWorldPose  sampleTime=0.01  busName='Gazebo_SL_Bus_gazebo_msgs_SetLinkWorldPose'
      settings: SourceProductBaseCode=RO
  Gazebo Select Entity : robotgazebolib/Gazebo Select Entity  modelElemName=ingenuity/leg3  outputArraySize=128  OutputLabel=Link  SelectType=Link
      settings: SourceProductBaseCode=RO
  Out1 : Outport
  wires:
  In6/1 -> Bus Assignment/9
  In4/1 -> Bus Assignment/7
  In3/1 -> Bus Assignment/6
  In7/1 -> Bus Assignment/10
  In2/1 -> Bus Assignment/5
  Bus Assignment/1 -> Out1/1
  Gazebo Select Entity/2 -> Bus Assignment/3
  In5/1 -> Bus Assignment/8
  Gazebo Blank Message/1 -> Bus Assignment/1
  In8/1 -> Bus Assignment/11
  In1/1 -> Bus Assignment/4
  Gazebo Select Entity/1 -> Bus Assignment/2

== system MARS/Gazebo Simulation/Link Body3 ==
  In1 : Inport
  In2 : Inport  Port=2
  In3 : Inport  Port=3
  In4 : Inport  Port=4
  In5 : Inport  Port=5
  In6 : Inport  Port=6
  In7 : Inport  Port=7
  In8 : Inport  Port=8
  Bus Assignment : BusAssignment  AssignedSignals=model_name,link_name,world_pose.position.x,world_pose.position.y,world_pose.position.z,world_pose.orientation.w,world_pose.orientation.x,world_pose.orientation.y,world_pose.orientation.z,duration.seconds
  Gazebo Blank Message : robotgazebolib/Gazebo Blank Message  msgType=SetLinkWorldPose  sampleTime=0.01  busName='Gazebo_SL_Bus_gazebo_msgs_SetLinkWorldPose'
      settings: SourceProductBaseCode=RO
  Gazebo Select Entity : robotgazebolib/Gazebo Select Entity  modelElemName=ingenuity/collective2  outputArraySize=128  OutputLabel=Link  SelectType=Link
      settings: SourceProductBaseCode=RO
  Out1 : Outport
  wires:
  Gazebo Select Entity/1 -> Bus Assignment/2
  In1/1 -> Bus Assignment/4
  In8/1 -> Bus Assignment/11
  Gazebo Blank Message/1 -> Bus Assignment/1
  In5/1 -> Bus Assignment/8
  Gazebo Select Entity/2 -> Bus Assignment/3
  Bus Assignment/1 -> Out1/1
  In2/1 -> Bus Assignment/5
  In7/1 -> Bus Assignment/10
  In3/1 -> Bus Assignment/6
  In4/1 -> Bus Assignment/7
  In6/1 -> Bus Assignment/9

== system MARS/Gazebo Simulation/Link Body4 ==
  In1 : Inport
  In2 : Inport  Port=2
  In3 : Inport  Port=3
  In4 : Inport  Port=4
  In5 : Inport  Port=5
  In6 : Inport  Port=6
  In7 : Inport  Port=7
  In8 : Inport  Port=8
  Bus Assignment : BusAssignment  AssignedSignals=model_name,link_name,world_pose.position.x,world_pose.position.y,world_pose.position.z,world_pose.orientation.w,world_pose.orientation.x,world_pose.orientation.y,world_pose.orientation.z,duration.seconds
  Gazebo Blank Message : robotgazebolib/Gazebo Blank Message  msgType=SetLinkWorldPose  sampleTime=0.01  busName='Gazebo_SL_Bus_gazebo_msgs_SetLinkWorldPose'
      settings: SourceProductBaseCode=RO
  Gazebo Select Entity : robotgazebolib/Gazebo Select Entity  modelElemName=ingenuity/leg2  outputArraySize=128  OutputLabel=Link  SelectType=Link
      settings: SourceProductBaseCode=RO
  Out1 : Outport
  wires:
  In6/1 -> Bus Assignment/9
  In4/1 -> Bus Assignment/7
  In3/1 -> Bus Assignment/6
  In7/1 -> Bus Assignment/10
  In2/1 -> Bus Assignment/5
  Bus Assignment/1 -> Out1/1
  Gazebo Select Entity/2 -> Bus Assignment/3
  In5/1 -> Bus Assignment/8
  Gazebo Blank Message/1 -> Bus Assignment/1
  In8/1 -> Bus Assignment/11
  In1/1 -> Bus Assignment/4
  Gazebo Select Entity/1 -> Bus Assignment/2

== system MARS/Gazebo Simulation/Link Body5 ==
  In1 : Inport
  In2 : Inport  Port=2
  In3 : Inport  Port=3
  In4 : Inport  Port=4
  In5 : Inport  Port=5
  In6 : Inport  Port=6
  In7 : Inport  Port=7
  In8 : Inport  Port=8
  Bus Assignment : BusAssignment  AssignedSignals=model_name,link_name,world_pose.position.x,world_pose.position.y,world_pose.position.z,world_pose.orientation.w,world_pose.orientation.x,world_pose.orientation.y,world_pose.orientation.z,duration.seconds
  Gazebo Blank Message : robotgazebolib/Gazebo Blank Message  msgType=SetLinkWorldPose  sampleTime=0.01  busName='Gazebo_SL_Bus_gazebo_msgs_SetLinkWorldPose'
      settings: SourceProductBaseCode=RO
  Gazebo Select Entity : robotgazebolib/Gazebo Select Entity  modelElemName=ingenuity/leg1  outputArraySize=128  OutputLabel=Link  SelectType=Link
      settings: SourceProductBaseCode=RO
  Out1 : Outport
  wires:
  Gazebo Select Entity/1 -> Bus Assignment/2
  In1/1 -> Bus Assignment/4
  In8/1 -> Bus Assignment/11
  Gazebo Blank Message/1 -> Bus Assignment/1
  In5/1 -> Bus Assignment/8
  Gazebo Select Entity/2 -> Bus Assignment/3
  Bus Assignment/1 -> Out1/1
  In2/1 -> Bus Assignment/5
  In7/1 -> Bus Assignment/10
  In3/1 -> Bus Assignment/6
  In4/1 -> Bus Assignment/7
  In6/1 -> Bus Assignment/9

== system MARS/Gazebo Simulation/Link Body6 ==
  In1 : Inport
  In2 : Inport  Port=2
  In3 : Inport  Port=3
  In4 : Inport  Port=4
  In5 : Inport  Port=5
  In6 : Inport  Port=6
  In7 : Inport  Port=7
  In8 : Inport  Port=8
  Bus Assignment : BusAssignment  AssignedSignals=model_name,link_name,world_pose.position.x,world_pose.position.y,world_pose.position.z,world_pose.orientation.w,world_pose.orientation.x,world_pose.orientation.y,world_pose.orientation.z,duration.seconds
  Gazebo Blank Message : robotgazebolib/Gazebo Blank Message  msgType=SetLinkWorldPose  sampleTime=0.01  busName='Gazebo_SL_Bus_gazebo_msgs_SetLinkWorldPose'
      settings: SourceProductBaseCode=RO
  Gazebo Select Entity : robotgazebolib/Gazebo Select Entity  modelElemName=ingenuity/collective1  outputArraySize=128  OutputLabel=Link  SelectType=Link
      settings: SourceProductBaseCode=RO
  Out1 : Outport
  wires:
  In6/1 -> Bus Assignment/9
  In4/1 -> Bus Assignment/7
  In3/1 -> Bus Assignment/6
  In7/1 -> Bus Assignment/10
  In2/1 -> Bus Assignment/5
  Bus Assignment/1 -> Out1/1
  Gazebo Select Entity/2 -> Bus Assignment/3
  In5/1 -> Bus Assignment/8
  Gazebo Blank Message/1 -> Bus Assignment/1
  In8/1 -> Bus Assignment/11
  In1/1 -> Bus Assignment/4
  Gazebo Select Entity/1 -> Bus Assignment/2

== system MARS/Gazebo Simulation/Link Body7 ==
  In1 : Inport
  In2 : Inport  Port=2
  In3 : Inport  Port=3
  In4 : Inport  Port=4
  In5 : Inport  Port=5
  In6 : Inport  Port=6
  In7 : Inport  Port=7
  In8 : Inport  Port=8
  Bus Assignment : BusAssignment  AssignedSignals=model_name,link_name,world_pose.position.x,world_pose.position.y,world_pose.position.z,world_pose.orientation.w,world_pose.orientation.x,world_pose.orientation.y,world_pose.orientation.z,duration.seconds
  Gazebo Blank Message : robotgazebolib/Gazebo Blank Message  msgType=SetLinkWorldPose  sampleTime=0.01  busName='Gazebo_SL_Bus_gazebo_msgs_SetLinkWorldPose'
      settings: SourceProductBaseCode=RO
  Gazebo Select Entity : robotgazebolib/Gazebo Select Entity  modelElemName=ingenuity/rotor1  outputArraySize=128  OutputLabel=Link  SelectType=Link
      settings: SourceProductBaseCode=RO
  Out1 : Outport
  wires:
  Gazebo Select Entity/1 -> Bus Assignment/2
  In1/1 -> Bus Assignment/4
  In8/1 -> Bus Assignment/11
  Gazebo Blank Message/1 -> Bus Assignment/1
  In5/1 -> Bus Assignment/8
  Gazebo Select Entity/2 -> Bus Assignment/3
  Bus Assignment/1 -> Out1/1
  In2/1 -> Bus Assignment/5
  In7/1 -> Bus Assignment/10
  In3/1 -> Bus Assignment/6
  In4/1 -> Bus Assignment/7
  In6/1 -> Bus Assignment/9

== system MARS/Gazebo Simulation/Link Body8 ==
  In1 : Inport
  In2 : Inport  Port=2
  In3 : Inport  Port=3
  In4 : Inport  Port=4
  In5 : Inport  Port=5
  In6 : Inport  Port=6
  In7 : Inport  Port=7
  In8 : Inport  Port=8
  Bus Assignment : BusAssignment  AssignedSignals=model_name,link_name,world_pose.position.x,world_pose.position.y,world_pose.position.z,world_pose.orientation.w,world_pose.orientation.x,world_pose.orientation.y,world_pose.orientation.z,duration.seconds
  Gazebo Blank Message : robotgazebolib/Gazebo Blank Message  msgType=SetLinkWorldPose  sampleTime=0.01  busName='Gazebo_SL_Bus_gazebo_msgs_SetLinkWorldPose'
      settings: SourceProductBaseCode=RO
  Gazebo Select Entity : robotgazebolib/Gazebo Select Entity  modelElemName=ingenuity/body  outputArraySize=128  OutputLabel=Link  SelectType=Link
      settings: SourceProductBaseCode=RO
  Out1 : Outport
  wires:
  In6/1 -> Bus Assignment/9
  In4/1 -> Bus Assignment/7
  In3/1 -> Bus Assignment/6
  In7/1 -> Bus Assignment/10
  In2/1 -> Bus Assignment/5
  Bus Assignment/1 -> Out1/1
  Gazebo Select Entity/2 -> Bus Assignment/3
  In5/1 -> Bus Assignment/8
  Gazebo Blank Message/1 -> Bus Assignment/1
  In8/1 -> Bus Assignment/11
  In1/1 -> Bus Assignment/4
  Gazebo Select Entity/1 -> Bus Assignment/2

== system MARS/Gazebo Simulation/Link Body9 ==
  In1 : Inport
  In2 : Inport  Port=2
  In3 : Inport  Port=3
  In4 : Inport  Port=4
  In5 : Inport  Port=5
  In6 : Inport  Port=6
  In7 : Inport  Port=7
  In8 : Inport  Port=8
  Bus Assignment : BusAssignment  AssignedSignals=model_name,link_name,world_pose.position.x,world_pose.position.y,world_pose.position.z,world_pose.orientation.w,world_pose.orientation.x,world_pose.orientation.y,world_pose.orientation.z,duration.seconds
  Gazebo Blank Message : robotgazebolib/Gazebo Blank Message  msgType=SetLinkWorldPose  sampleTime=0.01  busName='Gazebo_SL_Bus_gazebo_msgs_SetLinkWorldPose'
      settings: SourceProductBaseCode=RO
  Gazebo Select Entity : robotgazebolib/Gazebo Select Entity  modelElemName=ingenuity/leg4  outputArraySize=128  OutputLabel=Link  SelectType=Link
      settings: SourceProductBaseCode=RO
  Out1 : Outport
  wires:
  Gazebo Select Entity/1 -> Bus Assignment/2
  In1/1 -> Bus Assignment/4
  In8/1 -> Bus Assignment/11
  Gazebo Blank Message/1 -> Bus Assignment/1
  In5/1 -> Bus Assignment/8
  Gazebo Select Entity/2 -> Bus Assignment/3
  Bus Assignment/1 -> Out1/1
  In2/1 -> Bus Assignment/5
  In7/1 -> Bus Assignment/10
  In3/1 -> Bus Assignment/6
  In4/1 -> Bus Assignment/7
  In6/1 -> Bus Assignment/9

== system MARS/Gazebo Simulation/Rot2Quat ==
  "R1, R2, R3" : Inport
  Demux : Demux
  Rate w : RateTransition
  Rate x : RateTransition
  Rate y : RateTransition
  Rate z : RateTransition
  Rotation Angles to Quaternions : sharedtransform/Rotation Angles to Quaternions  rotationOrder=XYZ  aMode=aMode
      settings: SourceProductBaseCode=AE,PW,DR,MT,VE
  Out1 : Outport
  Out2 : Outport  Port=2
  Out3 : Outport  Port=3
  Out4 : Outport  Port=4
  wires:
  Demux/3 -> Rate y/1
  Demux/2 -> Rate x/1
  Demux/1 -> Rate w/1
  Demux/4 -> Rate z/1
  Rate x/1 -> Out2/1
  Rotation Angles to Quaternions/1 -> Demux/1
  "R1, R2, R3"/1 -> Rotation Angles to Quaternions/1
  Rate y/1 -> Out3/1
  Rate w/1 -> Out1/1
  Rate z/1 -> Out4/1

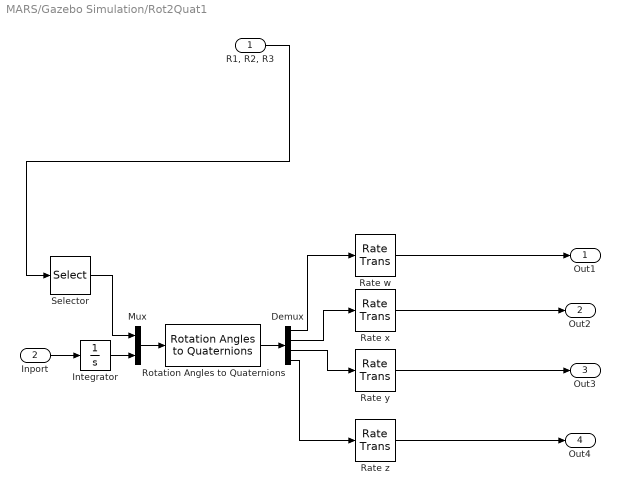
== system MARS/Gazebo Simulation/Rot2Quat1 ==
  "R1, R2, R3" : Inport
  Inport : Inport  Port=2
  Demux : Demux
  Integrator : Integrator
  Mux : Mux  Inputs=2
  Rate w : RateTransition
  Rate x : RateTransition
  Rate y : RateTransition
  Rate z : RateTransition
  Rotation Angles to Quaternions : sharedtransform/Rotation Angles to Quaternions  rotationOrder=XYZ  aMode=aMode
      settings: SourceProductBaseCode=AE,PW,DR,MT,VE
  Selector : Selector  InputPortWidth=3  IndexOptions=Index vector (dialog)  Indices=[1 2]  OutputSizes=1
  Out1 : Outport
  Out2 : Outport  Port=2
  Out3 : Outport  Port=3
  Out4 : Outport  Port=4
  wires:
  Rate z/1 -> Out4/1
  Rate w/1 -> Out1/1
  Rate y/1 -> Out3/1
  Rotation Angles to Quaternions/1 -> Demux/1
  Rate x/1 -> Out2/1
  Demux/4 -> Rate z/1
  Demux/1 -> Rate w/1
  Demux/2 -> Rate x/1
  Demux/3 -> Rate y/1
  Mux/1 -> Rotation Angles to Quaternions/1
  Selector/1 -> Mux/1
  "R1, R2, R3"/1 -> Selector/1
  Integrator/1 -> Mux/2
  Inport/1 -> Integrator/1

== system MARS/Gazebo Simulation/xyz ==
  In1 : Inport
  Demux1 : Demux  Outputs=3
  Rate Transition : RateTransition
  Rate Transition1 : RateTransition
  Rate Transition2 : RateTransition
  Out1 : Outport
  Out2 : Outport  Port=2
  Out3 : Outport  Port=3
  wires:
  Demux1/3 -> Rate Transition2/1
  Demux1/1 -> Rate Transition/1
  Demux1/2 -> Rate Transition1/1
  In1/1 -> Demux1/1
  Rate Transition/1 -> Out1/1
  Rate Transition1/1 -> Out2/1
  Rate Transition2/1 -> Out3/1

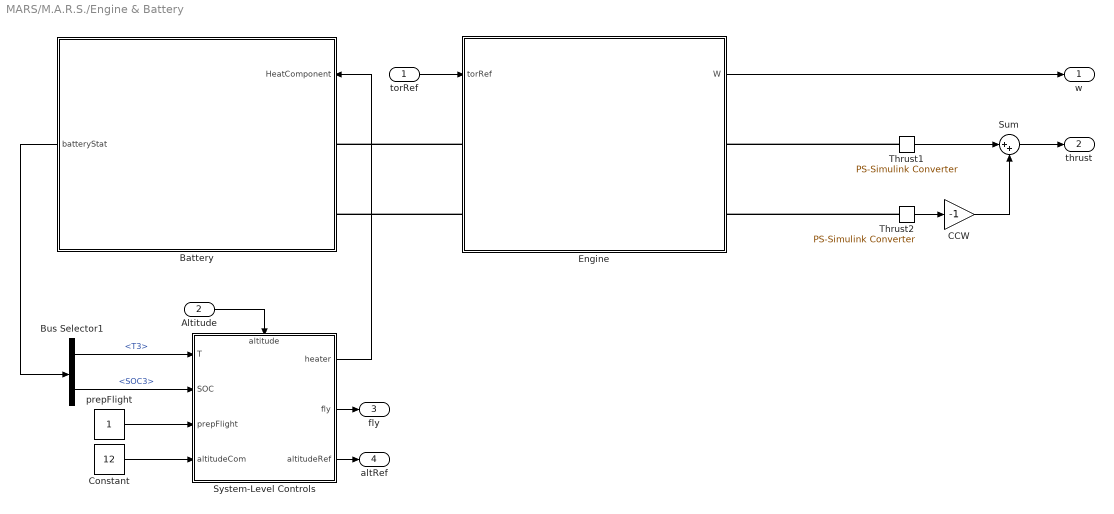
== system MARS/M.A.R.S./Engine & Battery ==
  torRef : Inport
  Altitude : Inport  Port=2
  Battery : Subsystem
      mask Display: image('$imagefile'); % Use "Edit Image" on toolstrip to change.
  Bus Selector1 : BusSelector  OutputSignals=T3,SOC3
  CCW : Gain  Gain=-1
  Constant : Constant  Value=12
  Engine : Subsystem
      mask Display: image('$imagefile'); % Use "Edit Image" on toolstrip to change.
  Sum : Sum  Inputs=|++
  System-Level Controls : Stateflow chart  TreatAsAtomicUnit=on
      settings: PortSchema="{\"entries\":[{\"content\":{\"sides\":[{\"content\":{\"connectorIds\":[\"In2\",\"In3\",\"In4\",\"In1\"]},\"type\":\"ConnectorPlacement.EquallySpacedRectSide\",\"uuid\":\"5067341e-d12a-4a2a-9253-3fb06d0079cf\"},{\"content\":{\"connectorIds\":[\"Out1\",\"Out2\",\"Out3\"],\"side\":\"RIGHT\"},\"type\":\"ConnectorPlacement.EquallySpacedRectSide\",\"uuid\":\"5404e1d9-f923-45fb-998d-e24e5a5fd6b6\"},{\"content\":{\"connectorIds\":[\"In5\"],\"side\":\"TOP\"},\"type\":\"ConnectorPlacement.EquallySpacedRectSide\",\"uuid\":\"b72b8578-46c7-4b5e-a689-fe24a80a6d63\"}]},\"type\":\"ConnectorPlacement.EquallySpacedConnector\",\"uuid\":\"f5827d07-5d2a-4259-8e8b-6d4ada56c462\"}],\"packageUris\":[\"http://schema.mathworks.com/mf0/Connector/R2020b\"],\"version\":\"1.0\"}"
  Thrust1 : nesl_utility/PS-Simulink Converter  PhysicalDomain=network_engine_domain  SubClassName=ps_output  LeftPortType=input  RightPortType=output  PseudoPeriodic=off  Frequencies=[]  VectorFormat=inherit  Unit=inherit  AffineConversion=off
      settings: SourceProductBaseCode=SS,PW,VE
  Thrust2 : nesl_utility/PS-Simulink Converter  PhysicalDomain=network_engine_domain  SubClassName=ps_output  LeftPortType=input  RightPortType=output  PseudoPeriodic=off  Frequencies=[]  VectorFormat=inherit  Unit=inherit  AffineConversion=off
      settings: SourceProductBaseCode=SS,PW,VE
  prepFlight : Constant
  w : Outport
  thrust : Outport  Port=2
  fly : Outport  Port=3
  altRef : Outport  Port=4
  wires:
  Thrust2/1 -> CCW/1
  Sum/1 -> thrust/1
  System-Level Controls/1(heater) -> Battery/1(HeatComponent)
  Battery/1(batteryStat) -> Bus Selector1/1
  System-Level Controls/2(fly) -> fly/1
  Bus Selector1/2 -> System-Level Controls/3(SOC)  "<SOC3>"
  Bus Selector1/1 -> System-Level Controls/2(T)  "<T3>"
  System-Level Controls/3(altitudeRef) -> altRef/1
  prepFlight/1 -> System-Level Controls/4(prepFlight)
  Altitude/1 -> System-Level Controls/5(altitude)
  Constant/1 -> System-Level Controls/1(altitudeCom)
  Thrust1/1 -> Sum/1
  CCW/1 -> Sum/2
  torRef/1 -> Engine/1(torRef)
  Engine/1(W) -> w/1
  connections:
  Thrust1/LConn1 -- Engine/RConn1
  Engine/LConn1 -- Battery/LConn1
  Engine/LConn2 -- Battery/LConn2
  Thrust2/LConn1 -- Engine/RConn2
